simulink model "Sim_Unknown_Constant_Gain_simtest"  (Simulink 7.3)
settings: Solver=VariableStepDiscrete  StartTime=0.0  StopTime=10.0  RelTol=1e-3
settings Model: Creator=MD710  LastModifiedBy=MD710
settings DebuggingCC: SaveWithParameterizedLinksMsg=none  SolverPrmCheckMsg=none  MultiTaskDSMMsg=warning  MultiTaskCondExecSysMsg=none  FcnCallInpInsideContextMsg=Enable All  StrictBusMsg=None
settings HardwareCC: TargetHWDeviceType=32-bit Generic
settings RTWCC: IncludeERTFirstTime=on
settings GRTTargetCC: TargetFcnLib=ansi_tfl_tmw.mat

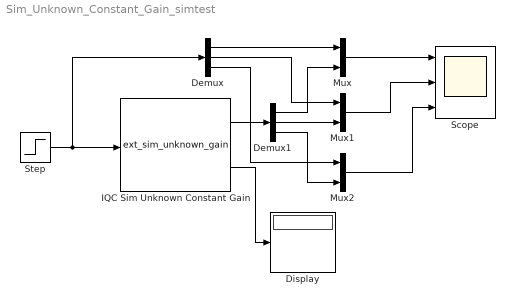
== system Sim_Unknown_Constant_Gain_simtest ==
  Demux : Demux  Outputs=3
  Demux1 : Demux  Outputs=3
  Display : Display
  IQC Sim Unknown Constant Gain : M-S-Function  FunctionName=ext_sim_unknown_gain  Parameters=sou_con,num_ran,cus,iqc1,iqc1_pole,iqc1_out,iqc2,iqc2_out,iqc3,iqc3_out,iqc4,lis_rel,rand_cons  mask(IQC Sim Unknown Constant Gain(ver:0.1)){sou_con=Random, num_ran=3, cus=[0], iqc1=on, iqc1_pole=[1], iqc1_out='', iqc2=off, iqc2_out='', iqc3=off, iqc3_out='', iqc4=off, lis_rel='', rand_cons=0}
      mask prompts: sou_con "Source of The Constant Gain:(Default: Random)"; num_ran "The Number of Random:(1 or input_dim)"; cus "Custom:"; iqc1 "iqc_ltigain(Input,Pole)"; iqc1_pole "Pole:(Default: [1])"; iqc1_out "Output Variable:(Default: empty)"; iqc2 "iqc_ltvnorm(Input,length(Input),1)"; iqc2_out "Output Variable:(Default: empty)"; iqc3 "iqc_tvscalar(Input,1)"; iqc3_out "Output Variable:(Default: empty)"; iqc4 "Custom IQC"; lis_rel "List of IQC Relationships:"; rand_cons "Mask Parameter 13:"
      mask init:
      | switch sou_con
      |     case 1
      |         rand_cons=rand(1,num_ran);
      |     case 2
      |         if any(abs(cus)>1)
      |             error('the maximum random constant is 1')
      |         else
      |             rand_cons=reshape(cus,1,length(cus));
      |         end
      | end
      mask Help:
      | <a href="matlab:doc iqc_ltigain;">iqc_ltigain</a>
      | <a href="matlab:doc iqc_ltvnorm;">iqc_ltvnorm</a>
      | <a href="matlab:doc iqc_tvscalar;">iqc_tvscalar</a>
      mask StyleString: popup(Random|Custom),edit,edit,checkbox,edit,edit,checkbox,edit,checkbox,edit,checkbox,edit,edit
      mask CallbackString: iqc_block_cho(gcb,'sim_constantgain_sou')|||iqc_block_cho(gcb,'sim_constantgain_iqc1')|||iqc_block_cho(gcb,'sim_constantgain_iqc2')||iqc_block_cho(gcb,'sim_constantgain_iqc3')||iqc_block_cho(gcb,'sim_constantgain_iqc4')||
      mask TabNameString: Simulink Parameters,Simulink Parameters,Simulink Parameters,Procedure Parameters,Procedure Parameters,Procedure Parameters,Procedure Parameters,Procedure Parameters,Procedure Parameters,Procedure Parameters,Procedure Parameters,Procedure Parameters,Simulink Parameters
      mask Display: disp('\fontsize{14}|d| < 1', 'texmode','on');port_label('input',1,'in');port_label('output',1,'out');port_label('output',2,'|d|');
  Mux : Mux  Inputs=2
  Mux1 : Mux  Inputs=2
  Mux2 : Mux  Inputs=2
  Scope : Scope  NumInputPorts=3
      settings: YMin=-5~-5~-5  YMax=5~5~5
  Step : Step  Time=[1 2 3]  Before=[0 0 0]  After=[5 3 1]  SampleTime=0
  wires:
  Step/1 -> Demux/1, IQC Sim Unknown Constant Gain/1
  IQC Sim Unknown Constant Gain/2 -> Display/1
  IQC Sim Unknown Constant Gain/1 -> Demux1/1
  Demux/1 -> Mux/1
  Demux1/1 -> Mux/2
  Mux/1 -> Scope/1
  Demux1/2 -> Mux1/2
  Demux/2 -> Mux1/1
  Mux1/1 -> Scope/2
  Demux/3 -> Mux2/1
  Demux1/3 -> Mux2/2
  Mux2/1 -> Scope/3
